simulink model "test3"  (Simulink 6.4)
settings: Solver=ode45  StartTime=0.0  StopTime=10.0  RelTol=1e-3
PreLoadFcn:
  | if exist('tl_preloadfcn','file'), tl_preloadfcn(gcs,95); end
PostLoadFcn:
  | if exist('tl_postloadfcn','file'), tl_postloadfcn(gcs,95); end
InitFcn:
  | if exist('tlds_start','file'), tlds_start(gcs); end
libraries: tllib x4
PreSaveFcn:
  | if exist('tl_presavefcn','file'), tl_presavefcn(gcs); end
settings Model: LastModifiedBy=alexh  TL_MAIN_DATA=struct('date',733386.55332849536,'maxnumsimulations',10,'codeopt',struct('inliningthreshold',6,'target',['Generic ANSI-C'],'assembler',0,'optlevel',2,'linebreaklimit',100,'stateactcodinglimit',5,'functionsfor64bitops',1,'sections',1,'sfbitfields',1,'globalbitfields',0,'sharefunctions',0,'noinitstozero',0,'limidentlength',1,'decimals',1,'separatesearch',0,'cleancode',0,'optimizedbooltype',1,'keepsaturation',0,'extvarsharing',0,'outputstylefile','cconfig.xml','rootstylesheet','TL_CSourceCodeSS.xsl','addchecksum',0,'modelsaving',2,'browsecodegen',0),'frameopt',struct('exectime',1,'stacksize',1,'simconfig',['default EVM'],'targettimeout',1,'mexargs','-g','tcargs',''),'logopt',struct('plotinterval',0.1,'globalloggingmode',1),'export',struct('directory','.\export','sysfiles',1,'docfiles',0,'tools',0),'codecoveragelevel',0,'asapscript','asap2_all_in_one','docscript','tldoc_default','rtos',struct('enablemultirate',0,'currentrtos',['generic RTOS'],'autopriority',0,'autoinitalarm',1,'alarminitwithrestart',1,'alarmactivationkind',1,'alarmstartoffset',0))  DS_PROJECTFILE=test3.dd

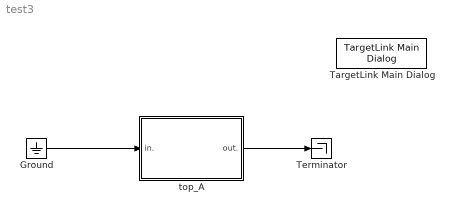
== system test3 ==
  Ground : Ground
  TargetLink Main Dialog : tllib/TargetLink Main Dialog  SystemSampleTime=-1  flp_block=none
  Terminator : Terminator
  top_A : Subsystem  Tag=TargetLink Simulation Frame
      settings: CopyFcn=if exist('tl_copyfcn','file'), tl_copyfcn(gcbh); end  NameChangeFcn=if exist('tl_framenamechangefcn','file'), tl_framenamechangefcn(gcbh); end  OpenFcn=if exist('open_tlsubsystem','file'), open_tlsubsystem(gcbh); end
      mask Type: TL_SimFrame
      mask Display: disp('TargetLink\nModel-\nin-the-loop\nmode')
  wires:
  top_A/1(out.) -> Terminator/1
  Ground/1 -> top_A/1(in.)

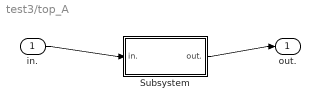
== system test3/top_A ==
  in. : Inport
  Subsystem : Subsystem  Tag=struct('sfcnName','top_A_sf','subFunction','','srcSubsystem','')
      settings: OpenFcn=warndlg(get_param(gcb,'MaskHelp'),'Serious Warning');
      mask Type: TL_Enable
      mask Help: This subsystem keeps the TargetLink subsystem (subsystem with TargetLink blocks for production code generation), and is needed for the TargetLink simulation frame to work properly. DO NOT DELETE OR MODIFY IT!
  out. : Outport
  wires:
  in./1 -> Subsystem/1(in.)
  Subsystem/1(out.) -> out./1

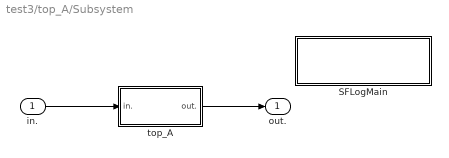
== system test3/top_A/Subsystem ==
  in. : Inport
  SFLogMain : Subsystem
      mask Type: TL_StateflowLoggingMain
      mask Display:
      | plot([0 0 1 1 0 0 1 1 0],[0 1 1 0 0 0.05 0.05 0.95 0.95]);
      | disp('Stateflow Logging Main\nDO NOT DELETE')
  top_A : Subsystem  Tag=MIL Subsystem  Description=a
      settings: CopyFcn=if exist('tl_copyfcn','file'), tl_copyfcn(gcbh); end  NameChangeFcn=if exist('tl_namechangefcn','file'), tl_namechangefcn(gcbh); end  DestroyFcn=if exist('update_tl_main_dlg','file'), update_tl_main_dlg('TL_subs_display'); end
  out. : Outport
  wires:
  in./1 -> top_A/1(in.)
  top_A/1(out.) -> out./1

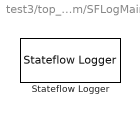
== system test3/top_A/Subsystem/SFLogMain ==
  Stateflow Logger : tllib/Extras/Stateflow Logger  data=struct('date',730486)  sflogparam=struct('charts',[],'sfblocks',[],'machines',[],'globallogopt',1,'modelname','test3','debugmodeactive',0)  flp_block=tldummylib/Stateflow Logger

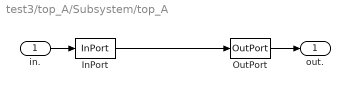
== system test3/top_A/Subsystem/top_A ==
  in. : Inport
      settings: CopyFcn=if exist('tl_check_ports','file'), tl_check_ports(gcbh); end  NameChangeFcn=if exist('tl_check_ports','file'), tl_check_ports(gcbh); end
  InPort : tllib/InPort  SystemSampleTime=-1  data=struct('logdata',struct('maxnumvals',inf,'plotchannels',[],'loggingmode',3,'channels',1),'output',struct('variable','','description','','name','$S_$B','width',1,'address','','max',NaN,'min',NaN,'class','OSC_VariableClassGroup/OSC_ES_GLOBAL','type','Int16','scaling','','lsb',1,'offset',0,'arb',0,'freeze',1,'unit','','autoscalingmode',1,'lowerheadroom',1,'upperheadroom',1,'headroomunit','bit','keepdatatype',1,'castoutput',0,'show',0),'inheritscaling',0,'message',struct('name','','component','','accessor',''),'virtual',1,'scalingvalid',0,'date',733386.6205014236)  flp_block=none
  OutPort : tllib/OutPort  SystemSampleTime=-1  data=struct('comment',struct('text','','placement',1),'logdata',struct('maxnumvals',inf,'plotchannels',[],'loggingmode',3,'channels',1),'output',struct('variable','','description','','name','$S_$B','width',1,'address','','max',NaN,'min',NaN,'class','default','type','Int16','scaling','','lsb',1,'offset',0,'arb',0,'freeze',1,'unit','','autoscalingmode',1,'lowerheadroom',1,'upperheadroom',1,'headroomunit','bit','keepdatatype',1,'checkmin',0,'checkmax',0,'castoutput',0,'show',0),'inheritscaling',0,'message',struct('name','','component',''),'virtual',1,'scalingvalid',0,'date',730486)  flp_block=none
  out. : Outport  InitialOutput=0
      settings: CopyFcn=if exist('tl_check_ports','file'), tl_check_ports(gcbh); end  NameChangeFcn=if exist('tl_check_ports','file'), tl_check_ports(gcbh); end
  wires:
  OutPort/1 -> out./1
  in./1 -> InPort/1
  InPort/1 -> OutPort/1
